simulink model "EMT_load"  (R2024a)
settings: Solver=ode1  StartTime=0.0  StopTime=simtime  FixedStep=Ts  RelTol=1e-3
values from neighbouring files (symbols this model uses):
  c0 = c0_hawk    (= 6.37282e-09)    [EMT_Phasor_parameters.m]
  c1 = c1_hawk    (= 8.76156e-09)    [EMT_Phasor_parameters.m]
  fg = 50    [EMT_Phasor_parameters.m]
  G1gen = 0.1245    [EMT_Phasor_parameters.m]
  G2gen = 0.30    (= 0.3)    [EMT_Phasor_parameters.m]
  G3gen = 0.20    (= 0.2)    [EMT_Phasor_parameters.m]
  G4sgen = 0.2078    [EMT_Phasor_parameters.m]
  G5gen = 0.20    (= 0.2)    [EMT_Phasor_parameters.m]
  G6gen = 0.2078    [EMT_Phasor_parameters.m]
  G6sgen = 0.20    (= 0.2)    [EMT_Phasor_parameters.m]
  G7gen = 0.518    [EMT_Phasor_parameters.m]
  Ihvpk = Ihv*sqrt(2)    [EMT_Phasor_parameters.m]
  l0 = l0_hawk    (= 0.00373)    [EMT_Phasor_parameters.m]
  l1 = l1_hawk    (= 0.00133)    [EMT_Phasor_parameters.m]
  L3dem = 0.10    (= 0.1)    [EMT_Phasor_parameters.m]
  L4dem = 0.30    (= 0.3)    [EMT_Phasor_parameters.m]
  L5dem = 0.35    [EMT_Phasor_parameters.m]
  L6dem = 0.15    [EMT_Phasor_parameters.m]
  L7dem = 0.10    (= 0.1)    [EMT_Phasor_parameters.m]
  Pr = Sr*PF    (= 550050000)    [EMT_Phasor_parameters.m]
  Qr = sqrt(Sr^2 - Pr^2)    [EMT_Phasor_parameters.m]
  r0 = r0_hawk    (= 0.44587)    [EMT_Phasor_parameters.m]
  r1 = r1_hawk    (= 0.12087)    [EMT_Phasor_parameters.m]
  Rtpu = Xtpu/40    (= 0.00375)    [EMT_Phasor_parameters.m]
  S1non = 400e6    (= 400000000)    [EMT_Phasor_parameters.m]
  S2non = 300e6    (= 300000000)    [EMT_Phasor_parameters.m]
  S3non = 200e6    (= 200000000)    [EMT_Phasor_parameters.m]
  S4snon = 200e6    (= 200000000)    [EMT_Phasor_parameters.m]
  S5non = 500e6    (= 500000000)    [EMT_Phasor_parameters.m]
  S6non = 400e6    (= 400000000)    [EMT_Phasor_parameters.m]
  S6snon = 200e6    (= 200000000)    [EMT_Phasor_parameters.m]
  S7non = 200e6    (= 200000000)    [EMT_Phasor_parameters.m]
  simtime = 5    [EMT_Phasor_parameters.m]
  tonvsc = 0.01    [EMT_Phasor_parameters.m]
  Ts = 150e-6    (= 0.00015)    [EMT_Phasor_parameters.m]
  Vhv = 220e3    (= 220000)    [EMT_Phasor_parameters.m]
  Vmv = 22e3    (= 22000)    [EMT_Phasor_parameters.m]
  wc1 = wsw1/10    (= 848.230016469)    [EMT_Phasor_parameters.m]
  wdc1 = wc1/10    (= 84.8230016469)    [EMT_Phasor_parameters.m]
  wpq1 = wc1/10    (= 84.8230016469)    [EMT_Phasor_parameters.m]
  wsw1 = ksw1*2*pi*fg    (= 8482.30016469)    [EMT_Phasor_parameters.m]
  Xtpu = 0.15    [EMT_Phasor_parameters.m]
undefined symbols (not defined in the file or in its folder): D11, Delta, Kf, r, theta0
libraries: simulink_extras x152, spsGroundLib x49, spsCurrentMeasurementLib x39, spsVoltageMeasurementLib x33, simulink x32, eeGeneralControl x32, slpidlib x32, powerlib x30, powerlib_meascontrol x28, spsFirstOrderFilterLib x24, eeTransforms x24, pid_lib x16
(part 6 of 16)

== system EMT_load/G2/VSC/VSC Control/Control loops/SW, EMT AVG, Phasor Quasi-EMT ==
  Pset : Inport
  Qset : Inport  Port=2
  vqd+- : Inport  Port=3
  iqd+- : Inport  Port=4
  freq : Inport  Port=5
  Block : Inport  Port=6
  Inner-loop : Subsystem
      settings: PortSchema="{\"entries\":[{\"content\":{\"sides\":[{\"content\":{\"connectorIds\":[\"In1\",\"In2\",\"In3\",\"In4\"]},\"type\":\"ConnectorPlacement.EquallySpacedRectSide\",\"uuid\":\"8a2e5096-891c-4956-8b6b-4b283c05b7bc\"},{\"content\":{\"connectorIds\":[\"Out1\",\"Out2\",\"Out3\",\"Out4\"],\"side\":\"RIGHT\"},\"type\":\"ConnectorPlacement.EquallySpacedRectSide\",\"uuid\":\"b7af4d2f-ce3f-4dc6-8323-535c80ee1784\"},{\"content\":{\"connectorIds\":[\"In5\",\"In6\",\"In7\"],\"side\":\"TOP\"},\"type\":\"ConnectorPlacement.EquallySpacedRectSide\",\"uuid\":\"1131cb27-465f-45b8-a6a1-03893285239a\"},{\"content\":{\"connectorIds\":[],\"side\":\"BOTTOM\"},\"type\":\"ConnectorPlacement.EquallySpacedRectSide\",\"uuid\":\"c84e74f4-9dae-42a7-97b7-61f404019883\"}]},\"type\":\"ConnectorPlacement.EquallySpacedConnector\",\"uuid\":\"8a900364-1293-46a0-8824-7b0f85f5a81c\"}],\"packageUris\":[\"http://schema.mathworks.com/mf0/Connector/19700101\"],\"version\":\"1.0\"}"
  Mux : Mux
  Outer-loop : Subsystem
      settings: PortSchema="{\"entries\":[{\"content\":{\"sides\":[{\"content\":{\"connectorIds\":[\"In1\",\"In2\",\"In3\",\"In4\",\"In5\"]},\"type\":\"ConnectorPlacement.EquallySpacedRectSide\",\"uuid\":\"9a334ab0-c6a2-41fb-a6ec-750715335523\"},{\"content\":{\"connectorIds\":[\"Out1\",\"Out2\",\"Out3\",\"Out4\",\"Out5\"],\"side\":\"RIGHT\"},\"type\":\"ConnectorPlacement.EquallySpacedRectSide\",\"uuid\":\"d3309230-0110-441f-b944-3d5d4312a42e\"},{\"content\":{\"connectorIds\":[\"In6\"],\"side\":\"TOP\"},\"type\":\"ConnectorPlacement.EquallySpacedRectSide\",\"uuid\":\"012603a1-4678-4ae1-91f6-3e17a1c8130b\"}]},\"type\":\"ConnectorPlacement.EquallySpacedConnector\",\"uuid\":\"299866d5-057c-44fe-b725-733ff7b8fc12\"}],\"packageUris\":[\"http://schema.mathworks.com/mf0/Connector/19700101\"],\"version\":\"1.0\"}"
  vqd+-ref : Outport
  m : Outport  Port=2
  wires:
  Mux/1 -> vqd+-ref/1
  Inner-loop/4(vd-*) -> Mux/4
  Inner-loop/3(vq-*) -> Mux/3
  Inner-loop/2(vd+*) -> Mux/2
  Inner-loop/1(vq+*) -> Mux/1
  Outer-loop/4(id-*) -> Inner-loop/4(id-*)
  Pset/1 -> Outer-loop/1(Pset)
  Qset/1 -> Outer-loop/2(Qset)
  Outer-loop/5(m) -> m/1
  Outer-loop/3(iq-*) -> Inner-loop/3(iq-*)
  freq/1 -> Outer-loop/5(freq)
  iqd+-/1 -> Inner-loop/7(iqd+-), Outer-loop/4(iqd+-)
  Block/1 -> Inner-loop/5(Blk), Outer-loop/6(Blk)
  vqd+-/1 -> Inner-loop/6(vqd+-), Outer-loop/3(vqd+-)
  Outer-loop/2(id+*) -> Inner-loop/2(id+*)
  Outer-loop/1(iq+*) -> Inner-loop/1(iq+*)

== system EMT_load/G2/VSC/VSC Control/Measurements/EMT ==
  note: abc to dq transformation
  Vabc : Inport
  Iabc : Inport  Port=2
  Gain2 : Gain  Gain=Vmv/Vhv
  Gain3 : Gain  Gain=Vhv/Vmv
  Iabc filter : spsFirstOrderFilterLib/First-Order Filter  Commented=through  FilterType=Lowpass  Tc=tfilt  Ts=0  Initialize=off  Vac_Init=[0, 0, 60]  Vdc_Init=0  PlotResponse=off  FreqRange="[0,  200,  1]"
  Mux : Mux
  Mux2 : Mux
  Mux3 : Mux  Inputs=2
  PLL aligned with positive-sequence : Subsystem
  Phase-sequence separation2 : Subsystem
  Phase-sequence separation3 : Subsystem
  "Power (3ph, Instantaneous)" : spsPower3phInstantaneousLib/Power (3ph, Instantaneous)
  Vabc filter : spsFirstOrderFilterLib/First-Order Filter  Commented=through  FilterType=Lowpass  Tc=tfilt  Ts=0  Initialize=off  Vac_Init=[0, 0, 60]  Vdc_Init=0  PlotResponse=off  FreqRange="[0,  200,  1]"
  freq : Outport
  theta : Outport  Port=2
  vqd+- : Outport  Port=3
  iqd+- : Outport  Port=4
  PQabc : Outport  Port=5
  wires:
  Phase-sequence separation2/2(d+) -> Mux/2
  Phase-sequence separation2/1(q+) -> Mux/1
  Iabc filter/1 -> Gain3/1
  Gain2/1 -> PLL aligned with positive-sequence/1(Vabc), Phase-sequence separation2/1(abc)
  Gain3/1 -> Phase-sequence separation3/1(abc)
  PLL aligned with positive-sequence/1(theta) -> Phase-sequence separation3/2(Theta), theta/1, Phase-sequence separation2/2(Theta)  "theta"
  PLL aligned with positive-sequence/2(f) -> freq/1
  Iabc/1 -> Iabc filter/1, [Iabc]
  Vabc filter/1 -> Gain2/1
  Vabc/1 -> Vabc filter/1, [Vabc]
  Mux/1 -> vqd+-/1  "vqd+-"
  Mux2/1 -> iqd+-/1  "iqd+-"
  Phase-sequence separation2/3(q-) -> Mux/3
  Phase-sequence separation2/4(d-) -> Mux/4
  Phase-sequence separation3/1(q+) -> Mux2/1
  Phase-sequence separation3/2(d+) -> Mux2/2
  Phase-sequence separation3/3(q-) -> Mux2/3
  Phase-sequence separation3/4(d-) -> Mux2/4
  "Power (3ph, Instantaneous)"/2 -> Mux3/2
  "Power (3ph, Instantaneous)"/1 -> Mux3/1
  Mux3/1 -> PQabc/1  "PQ1"
  [Iabc] -> "Power (3ph, Instantaneous)"/2
  [Vabc] -> "Power (3ph, Instantaneous)"/1

== system EMT_load/G2/VSC/VSC Control/Measurements/Phasor ==
  note: abc to dq transformation
      | (Phasor)
  Vabc : Inport
  Iabc : Inport  Port=2
  Complex to Magnitude-Angle : ComplexToMagnitudeAngle  Output=Angle
  Complex to Real-Imag{,1..3} (4 alike) : ComplexToRealImag
  Demux1 : Demux  Outputs=3
  Demux2 : Demux  Outputs=3
  Exp : Math  OutputSignalType=complex
  Frequency (Phasor)1 : Subsystem  mask{f0=fg, Ts=5e-3}
      mask prompts: f0 "Fundamental frequency (Hz)"; Ts "Derivative filter time constant (s)"
  Gain{,3..4,6..7} (5 alike) : Gain  Gain=-1
  Gain1 : Gain  Gain=Vhv/Vmv
  Gain2 : Gain  Gain=Vmv/Vhv
  Gain5 : Gain  Gain=-1i
  Instantaneous power (Phasor) : Subsystem
  Mux1 : Mux
  Mux2 : Mux
  Mux3 : Mux  Inputs=2
  Product{1..4} (4 alike) : Product
  Subsystem : Subsystem
      mask init:
      | a = exp(1i*2*pi/3);
      | a2 = exp(1i*4*pi/3);
  Subsystem1 : Subsystem
      mask init:
      | a = exp(1i*2*pi/3);
      | a2 = exp(1i*4*pi/3);
  Subsystem3 : Subsystem
      mask init:
      | a = exp(1i*2*pi/3);
      | a2 = exp(1i*4*pi/3);
  Terminator2 : Terminator
  Terminator4 : Terminator
  vqd+- : Outport
  iqd+- : Outport  Port=2
  freq : Outport  Port=3
  theta : Outport  Port=4
  PQabc : Outport  Port=5
  wires:
  Gain7/1 -> Mux2/4
  Gain6/1 -> Mux2/3
  Exp/1 -> Product1/1, Product4/1, Product2/2, Product3/2
  Product3/1 -> Complex to Real-Imag/1
  Demux2/2 -> Product3/1
  Demux2/3 -> Product2/1
  Gain5/1 -> Exp/1
  Complex to Magnitude-Angle/1 -> Frequency (Phasor)1/1(Phase), Gain5/1, theta/1  "theta"
  Product4/1 -> Complex to Real-Imag1/1
  Complex to Real-Imag/2 -> Mux1/2  "vd+"
  Demux1/3 -> Product1/2
  Demux1/2 -> Product4/2
  Subsystem/1(012) -> Demux2/1
  Demux2/1 -> Terminator2/1
  Demux1/1 -> Terminator4/1
  Subsystem1/1(012) -> Demux1/1
  Subsystem3/1(seq+) -> Complex to Magnitude-Angle/1
  Frequency (Phasor)1/1(Freq) -> freq/1
  Vabc/1 -> [Vabc], Gain2/1
  Gain2/1 -> Subsystem3/1(abc), Subsystem/1(abc)
  Product2/1 -> Complex to Real-Imag2/1
  Product1/1 -> Complex to Real-Imag3/1
  Mux1/1 -> vqd+-/1
  Complex to Real-Imag/1 -> Mux1/1  "vq+"
  Complex to Real-Imag2/1 -> Gain/1  "vq-"
  Complex to Real-Imag2/2 -> Gain3/1  "vd-"
  Complex to Real-Imag1/1 -> Mux2/1  "iq+"
  Complex to Real-Imag1/2 -> Gain4/1  "id+"
  Complex to Real-Imag3/1 -> Gain6/1  "iq-"
  Complex to Real-Imag3/2 -> Gain7/1  "id-"
  Mux2/1 -> iqd+-/1
  Iabc/1 -> [Iabc], Gain1/1
  Gain1/1 -> Subsystem1/1(abc)
  Gain/1 -> Mux1/3
  Gain3/1 -> Mux1/4
  Gain4/1 -> Mux2/2
  [Iabc] -> Instantaneous power (Phasor)/2(Iabc)
  Instantaneous power (Phasor)/2(Q) -> Mux3/2
  Instantaneous power (Phasor)/1(P) -> Mux3/1
  [Vabc] -> Instantaneous power (Phasor)/1(Vabc)
  Mux3/1 -> PQabc/1

== system EMT_load/G2/VSC/VSC Control/Modulation/EMT AVG ==
  note: Positive-sequence dq to abc
  note: Vref
  note: dq to abc
      | (AVG Model)
  note: negative-sequence dq to abc
  vqd+-* : Inport
  theta : Inport  Port=2
  Cartesian to Polar : simulink_extras/Transformations/Cartesian to Polar
  Cartesian to Polar1 : simulink_extras/Transformations/Cartesian to Polar
  Constant1 : Constant  Value=0
  Constant2 : Constant  Value=0
  Corrects delay : Subsystem
  Corrects delay1 : Subsystem
  Demux : Demux
  Gain : Gain  Gain=-1
  Gain2 : Gain  Gain=negseq_en
  Inverse Park Transform : eeTransforms/Inverse Park Transform  AxisAlignment=D-axis  PowerInvariant=off
  Inverse Park Transform1 : eeTransforms/Inverse Park Transform  AxisAlignment=D-axis  PowerInvariant=off
  Mux1 : Mux  Inputs=3
  Mux2 : Mux  Inputs=3
  Polar to Cartesian : simulink_extras/Transformations/Polar to Cartesian
  Polar to Cartesian1 : simulink_extras/Transformations/Polar to Cartesian
  Sum : Sum
  Sum1 : Sum  Inputs=|++
  Sum4 : Sum  Inputs=|++
  Unit Delay : UnitDelay  SampleTime=-1  HasFrameUpgradeWarning=on
  Ref : Outport
  wires:
  Demux/3 -> [vqnref]
  Demux/1 -> [vqpref]
  Demux/4 -> [vdnref]
  Demux/2 -> [vdpref]
  vqd+-*/1 -> Demux/1
  Gain2/1 -> Sum/2
  Polar to Cartesian/2 -> Mux1/2
  Sum4/1 -> Polar to Cartesian/2
  Mux1/1 -> Inverse Park Transform/1
  Cartesian to Polar/1 -> Polar to Cartesian/1
  [vdpref] -> Cartesian to Polar/1
  Cartesian to Polar/2 -> Sum4/1
  Constant1/1 -> Mux1/3
  [vqpref] -> Cartesian to Polar/2
  Corrects delay/1(dphi) -> Sum4/2
  Polar to Cartesian/1 -> Mux1/1
  Unit Delay/1 -> Ref/1
  [vdnref] -> Cartesian to Polar1/1
  Mux2/1 -> Inverse Park Transform1/1
  Cartesian to Polar1/1 -> Polar to Cartesian1/1
  Constant2/1 -> Mux2/3
  Polar to Cartesian1/2 -> Mux2/2
  Sum1/1 -> Polar to Cartesian1/2
  [vqnref] -> Cartesian to Polar1/2
  Corrects delay1/1(dphi) -> Sum1/2
  Gain/1 -> Inverse Park Transform1/2
  Polar to Cartesian1/1 -> Mux2/1
  Cartesian to Polar1/2 -> Sum1/1
  theta/1 -> Gain/1, Inverse Park Transform/2
  Sum/1 -> Unit Delay/1
  Inverse Park Transform/1 -> Sum/1
  Inverse Park Transform1/1 -> Gain2/1

== system EMT_load/G2/VSC/VSC Control/Modulation/EMT Switching ==
  note: Interpolate pulses
  note: Pulses
  note: Modulation
  note: negative-sequence dq to abc
  note: Positive-sequence dq to abc
  vqd+-* : Inport
  theta : Inport  Port=2
  Cartesian to Polar : simulink_extras/Transformations/Cartesian to Polar
  Cartesian to Polar1 : simulink_extras/Transformations/Cartesian to Polar
  Constant : Constant  Value=0
  Constant1 : Constant  Commented=on  Value=Vdc
  Constant2 : Constant  Value=0
  Corrects delay : Subsystem
  Corrects delay1 : Subsystem
  Demux : Demux
  Gain : Gain  Gain=1/(Vdc/2)
  Gain1 : Gain  Gain=-1
  Gain2 : Gain  Gain=negseq_en
  Inverse Park Transform1 : eeTransforms/Inverse Park Transform  AxisAlignment=D-axis  PowerInvariant=off
  Inverse Park Transform2 : eeTransforms/Inverse Park Transform  AxisAlignment=D-axis  PowerInvariant=off
  Mux : Mux  Inputs=3
  Mux1 : Mux  Inputs=3
  Mux2 : Mux  Inputs=3
  PWM Generator (Interpolation)1 : powerlib_meascontrol/Pulse & Signal Generators/PWM Generator (Interpolation)  GeneratorType=Two-level, three-phase  Fc=ksw*fg  InitialPhase=0  Ts=Ts
  "PWM Generator (Three-phase, Two-level)" : eePwmGeneratorTwoLevel/PWM Generator (Three-phase, Two-level)  Commented=on  PWMMode=Continuous PWM (CPWM)  CPWMMode=SPWM: sinusoidal PWM  DPWMMode=60 DPWM: 60 degree discontinuous PWM  fsw=ksw*fg  Ts=Ts
  Polar to Cartesian : simulink_extras/Transformations/Polar to Cartesian
  Polar to Cartesian1 : simulink_extras/Transformations/Polar to Cartesian
  Sum : Sum
  Sum1 : Sum  Inputs=|++
  Sum4 : Sum  Inputs=|++
  Unit Delay : UnitDelay  SampleTime=-1  HasFrameUpgradeWarning=on
  Ref : Outport
  wires:
  [vqpref] -> Cartesian to Polar/2
  Demux/4 -> [vdnref]
  Demux/3 -> [vqnref]
  Demux/2 -> [vdpref]
  Demux/1 -> [vqpref]
  vqd+-*/1 -> Demux/1
  Mux1/1 -> Unit Delay/1
  Sum/1 -> Gain/1
  Unit Delay/1 -> Ref/1
  PWM Generator (Interpolation)1/2 -> Mux1/2
  PWM Generator (Interpolation)1/1 -> Mux1/1
  PWM Generator (Interpolation)1/3 -> Mux1/3
  Gain/1 -> PWM Generator (Interpolation)1/1
  Constant1/1 -> "PWM Generator (Three-phase, Two-level)"/2
  theta/1 -> Inverse Park Transform2/2, Gain1/1
  Gain2/1 -> Sum/2
  Constant/1 -> Mux/3
  Cartesian to Polar/2 -> Sum4/1
  Sum4/1 -> Polar to Cartesian/2
  Corrects delay/1(dphi) -> Sum4/2
  Cartesian to Polar/1 -> Polar to Cartesian/1
  Mux/1 -> Inverse Park Transform2/1
  Polar to Cartesian/1 -> Mux/1
  Polar to Cartesian/2 -> Mux/2
  [vdpref] -> Cartesian to Polar/1
  Mux2/1 -> Inverse Park Transform1/1
  Sum1/1 -> Polar to Cartesian1/2
  Inverse Park Transform2/1 -> Sum/1
  Corrects delay1/1(dphi) -> Sum1/2
  Polar to Cartesian1/2 -> Mux2/2
  Cartesian to Polar1/1 -> Polar to Cartesian1/1
  Cartesian to Polar1/2 -> Sum1/1
  Polar to Cartesian1/1 -> Mux2/1
  [vdnref] -> Cartesian to Polar1/1
  [vqnref] -> Cartesian to Polar1/2
  Inverse Park Transform1/1 -> Gain2/1
  Constant2/1 -> Mux2/3
  Gain1/1 -> Inverse Park Transform1/2

== system EMT_load/G2/VSC/VSC Control/Modulation/Phasor I and Phasor PQ ==
  note: Negative-sequence dq to abc
  note: Positive-sequence dq to abc
  note: dq to abc
      | (Phasor I and Phasor PQ)
  iqd+-* : Inport
  theta : Inport  Port=2
  Constant : Constant  Commented=on  Value=negseq_en
  Constant1 : Constant  Value=complex(0,0)
  Delay : Delay  DelayLength=1
  Demux3 : Demux
  Display : Display  Commented=on
  Exp : Math  OutputSignalType=complex
  Exp1 : Math  OutputSignalType=complex
  Gain : Gain  Gain=-1
  Gain1 : Gain  Gain=1i
  Gain2 : Gain  Gain=exp(1i*pi/6)
  Gain3 : Gain  Gain=exp(-1i*pi/6)
  Gain5 : Gain  Gain=1i
  Gain7 : Gain  Gain=negseq_en
  Gain8 : Gain  Gain=-1
  Gain9 : Gain  Gain=-1
  Inverse Park Transform (Phasor) : Subsystem  Commented=on
  Mux3 : Mux  Inputs=3
  Product : Product
  Product1 : Product
  RL time constant : Subsystem  Commented=through  mask{R=Rt, L=Lt, f=fg}
      mask prompts: R "Series resistance (R)"; L "Series inductance (L)"; f "Power frequency (Hz)"
      mask init:
      | w = 2*pi*f;
  Real-Imag to Complex : RealImagToComplex
  Real-Imag to Complex1 : RealImagToComplex
  Subsystem : Subsystem
      mask init:
      | a = exp(1i*2*pi/3);
      | a2 = exp(1i*4*pi/3);
  Ref : Outport
  wires:
  Demux3/4 -> [idnref]
  iqd+-*/1 -> Demux3/1
  Demux3/1 -> [iqpref]
  Demux3/2 -> [idpref]
  Demux3/3 -> [iqnref]
  Constant/1 -> Display/1
  Gain/1 -> Real-Imag to Complex/2
  [idpref] -> Gain/1
  Exp1/1 -> Product1/1
  Real-Imag to Complex1/1 -> Product1/2
  Gain1/1 -> Exp1/1
  Constant1/1 -> Mux3/1
  Mux3/1 -> Subsystem/1(012)
  Product/1 -> Gain2/1
  Real-Imag to Complex/1 -> Product/1
  [iqpref] -> Real-Imag to Complex/1
  Exp/1 -> Product/2
  Gain5/1 -> Exp/1
  theta/1 -> Gain1/1, Gain5/1
  Delay/1 -> Ref/1
  Subsystem/1(abc) -> Delay/1
  Gain3/1 -> Mux3/3
  Product1/1 -> Gain7/1
  Gain7/1 -> Gain3/1
  [idnref] -> Gain8/1
  [iqnref] -> Gain9/1
  Gain9/1 -> Real-Imag to Complex1/1
  Gain8/1 -> Real-Imag to Complex1/2
  Gain2/1 -> Mux3/2

== system EMT_load/G2/VSC/VSC Control/Modulation/Phasor Quasi-EMT ==
  note: dq to abc
      | (Phasor)
  note: Positive-sequence dq to abc
  note: Negative-sequence dq to abc
  vqd+-* : Inport
  theta : Inport  Port=2
  vqd+- : Inport  Port=3
  Cartesian to Polar : simulink_extras/Transformations/Cartesian to Polar
  Cartesian to Polar1 : simulink_extras/Transformations/Cartesian to Polar
  Constant : Constant  Commented=on  Value=negseq_en
  Constant1 : Constant  Value=complex(0,0)
  Corrects delay : Subsystem  Commented=on
  Corrects delay2 : Subsystem  Commented=on
  Delay : Delay  DelayLength=1
  Demux : Demux  Outputs=2
  Demux1 : Demux  Outputs=2
  Demux2 : Demux
  Demux3 : Demux
  Display : Display  Commented=on
  Exp : Math  OutputSignalType=complex
  Exp1 : Math  OutputSignalType=complex
  Gain : Gain  Gain=-1
  Gain1 : Gain  Gain=1i
  Gain2 : Gain  Gain=exp(1i*pi/6)
  Gain3 : Gain  Gain=exp(-1i*pi/6)
  Gain5 : Gain  Gain=1i
  Gain7 : Gain  Gain=negseq_en
  Gain8 : Gain  Gain=-1
  Gain9 : Gain  Gain=-1
  Inverse Park Transform (Phasor) : Subsystem  Commented=on
  Mux{,1..2,4} (4 alike) : Mux  Inputs=2
  Mux3 : Mux  Inputs=3
  Polar to Cartesian : simulink_extras/Transformations/Polar to Cartesian
  Polar to Cartesian1 : simulink_extras/Transformations/Polar to Cartesian
  Product : Product
  Product1 : Product
  Real-Imag to Complex : RealImagToComplex
  Real-Imag to Complex1 : RealImagToComplex
  Subsystem : Subsystem
      mask init:
      | a = exp(1i*2*pi/3);
      | a2 = exp(1i*4*pi/3);
  Sum1 : Sum  Inputs=|++
  Sum4 : Sum  Inputs=|++
  V to I RL (+seq) : Subsystem  mask{R=Rt, L=Lt, f=fg}
      mask prompts: R "Series resistance (R)"; L "Series inductance (L)"; f "Power frequency (Hz)"
      mask init:
      | w = 2*pi*f;
  V to I RL (- seq) : Subsystem  mask{R=Rt, L=Lt, f=fg}
      mask prompts: R "Series resistance (R)"; L "Series inductance (L)"; f "Power frequency (Hz)"
      mask init:
      | w = 2*pi*f;
  Ref : Outport
  wires:
  Demux3/3 -> [vqnref]
  Demux3/4 -> [vdnref]
  Demux3/1 -> [vqpref]
  vqd+-*/1 -> Demux3/1
  Demux3/2 -> [vdpref]
  Gain2/1 -> Mux3/2
  Gain8/1 -> Real-Imag to Complex1/2
  Gain9/1 -> Real-Imag to Complex1/1
  Demux1/2 -> Gain9/1
  Demux1/1 -> Gain8/1
  Gain7/1 -> Gain3/1
  Product1/1 -> Gain7/1
  Gain3/1 -> Mux3/3
  Subsystem/1(abc) -> Delay/1
  Delay/1 -> Ref/1
  Cartesian to Polar1/1 -> Polar to Cartesian1/1
  theta/1 -> Gain5/1, Gain1/1
  [vqp] -> Mux1/2
  V to I RL (+seq)/1(idIq) -> Demux/1
  Gain5/1 -> Exp/1
  Exp/1 -> Product/2
  Demux/2 -> Real-Imag to Complex/1
  Real-Imag to Complex/1 -> Product/1
  Product/1 -> Gain2/1
  Mux3/1 -> Subsystem/1(012)
  Constant1/1 -> Mux3/1
  Sum4/1 -> Polar to Cartesian/2
  Cartesian to Polar/1 -> Polar to Cartesian/1
  Cartesian to Polar/2 -> Sum4/1
  Corrects delay/1(dphi) -> Sum4/2
  Polar to Cartesian/1 -> Mux/1
  Polar to Cartesian/2 -> Mux/2
  [vdpref] -> Cartesian to Polar/1
  [vqpref] -> Cartesian to Polar/2
  Mux/1 -> V to I RL (+seq)/2(Vdq2)
  Mux1/1 -> V to I RL (+seq)/1(Vdq1)
  [vdnref] -> Cartesian to Polar1/1
  Sum1/1 -> Polar to Cartesian1/2
  [vqnref] -> Cartesian to Polar1/2
  Polar to Cartesian1/2 -> Mux2/2
  Polar to Cartesian1/1 -> Mux2/1
  Cartesian to Polar1/2 -> Sum1/1
  Corrects delay2/1(dphi) -> Sum1/2
  Mux2/1 -> V to I RL (- seq)/2(Vdq2)
  Mux4/1 -> V to I RL (- seq)/1(Vdq1)
  [vqn] -> Mux4/2
  [vdn] -> Mux4/1
  V to I RL (- seq)/1(idIq) -> Demux1/1
  Gain1/1 -> Exp1/1
  Real-Imag to Complex1/1 -> Product1/2
  Exp1/1 -> Product1/1
  vqd+-/1 -> Demux2/1
  Demux2/2 -> [vdp]
  Demux2/3 -> [vqn]
  Demux2/4 -> [vdn]
  Demux2/1 -> [vqp]
  [vdp] -> Mux1/1
  Demux/1 -> Gain/1
  Gain/1 -> Real-Imag to Complex/2
  Constant/1 -> Display/1

== system EMT_load/G3/VSC/VSC Control/Control loops/Phasor I 1st ==
  Pset : Inport
  Qset : Inport  Port=2
  vqd+- : Inport  Port=3
  iqd+- : Inport  Port=4
  freq : Inport  Port=5
  Block : Inport  Port=6
  Inner-loop : Subsystem
  Mux : Mux
  Outer-loop : Subsystem
      settings: PortSchema="{\"entries\":[{\"content\":{\"sides\":[{\"content\":{\"connectorIds\":[\"In1\",\"In2\",\"In3\",\"In4\",\"In5\"]},\"type\":\"ConnectorPlacement.EquallySpacedRectSide\",\"uuid\":\"9a334ab0-c6a2-41fb-a6ec-750715335523\"},{\"content\":{\"connectorIds\":[\"Out1\",\"Out2\",\"Out3\",\"Out4\",\"Out5\"],\"side\":\"RIGHT\"},\"type\":\"ConnectorPlacement.EquallySpacedRectSide\",\"uuid\":\"d3309230-0110-441f-b944-3d5d4312a42e\"},{\"content\":{\"connectorIds\":[\"In6\"],\"side\":\"TOP\"},\"type\":\"ConnectorPlacement.EquallySpacedRectSide\",\"uuid\":\"012603a1-4678-4ae1-91f6-3e17a1c8130b\"}]},\"type\":\"ConnectorPlacement.EquallySpacedConnector\",\"uuid\":\"299866d5-057c-44fe-b725-733ff7b8fc12\"}],\"packageUris\":[\"http://schema.mathworks.com/mf0/Connector/19700101\"],\"version\":\"1.0\"}"
  iqd+-ref : Outport
  m : Outport  Port=2
  wires:
  Outer-loop/4(id-*) -> Inner-loop/4(id-*)
  Outer-loop/3(iq-*) -> Inner-loop/3(iq-*)
  Outer-loop/2(id+*) -> Inner-loop/2(id+*)
  Outer-loop/1(iq+*) -> Inner-loop/1(iq+*)
  Block/1 -> Outer-loop/6(Blk)
  vqd+-/1 -> Outer-loop/3(vqd+-)
  freq/1 -> Outer-loop/5(freq)
  iqd+-/1 -> Outer-loop/4(iqd+-)
  Inner-loop/2(id+ref) -> Mux/2
  Pset/1 -> Outer-loop/1(Pset)
  Outer-loop/5(m) -> m/1
  Qset/1 -> Outer-loop/2(Qset)
  Mux/1 -> iqd+-ref/1
  Inner-loop/3(iq-ref) -> Mux/3
  Inner-loop/1(iq+ref) -> Mux/1
  Inner-loop/4(id-ref) -> Mux/4

== system EMT_load/G3/VSC/VSC Control/Control loops/Phasor I ref ==
  Pset : Inport
  Qset : Inport  Port=2
  vqd+- : Inport  Port=3
  iqd+- : Inport  Port=4
  freq : Inport  Port=5
  Block : Inport  Port=6
  Mux : Mux
  Outer-loop : Subsystem
      settings: PortSchema="{\"entries\":[{\"content\":{\"sides\":[{\"content\":{\"connectorIds\":[\"In1\",\"In2\",\"In3\",\"In4\",\"In5\"]},\"type\":\"ConnectorPlacement.EquallySpacedRectSide\",\"uuid\":\"9a334ab0-c6a2-41fb-a6ec-750715335523\"},{\"content\":{\"connectorIds\":[\"Out1\",\"Out2\",\"Out3\",\"Out4\",\"Out5\"],\"side\":\"RIGHT\"},\"type\":\"ConnectorPlacement.EquallySpacedRectSide\",\"uuid\":\"d3309230-0110-441f-b944-3d5d4312a42e\"},{\"content\":{\"connectorIds\":[\"In6\"],\"side\":\"TOP\"},\"type\":\"ConnectorPlacement.EquallySpacedRectSide\",\"uuid\":\"012603a1-4678-4ae1-91f6-3e17a1c8130b\"}]},\"type\":\"ConnectorPlacement.EquallySpacedConnector\",\"uuid\":\"299866d5-057c-44fe-b725-733ff7b8fc12\"}],\"packageUris\":[\"http://schema.mathworks.com/mf0/Connector/19700101\"],\"version\":\"1.0\"}"
  iqd+-ref : Outport
  m : Outport  Port=2
  wires:
  Outer-loop/4(id-*) -> Mux/4
  Outer-loop/1(iq+*) -> Mux/1
  Outer-loop/3(iq-*) -> Mux/3
  Mux/1 -> iqd+-ref/1
  Qset/1 -> Outer-loop/2(Qset)
  Outer-loop/5(m) -> m/1
  Pset/1 -> Outer-loop/1(Pset)
  Outer-loop/2(id+*) -> Mux/2
  iqd+-/1 -> Outer-loop/4(iqd+-)
  freq/1 -> Outer-loop/5(freq)
  vqd+-/1 -> Outer-loop/3(vqd+-)
  Block/1 -> Outer-loop/6(Blk)

== system EMT_load/G3/VSC/VSC Control/Control loops/Phasor PQ 1st ==
  Pset : Inport
  Qset : Inport  Port=2
  vqd+- : Inport  Port=3
  iqd+- : Inport  Port=4
  freq : Inport  Port=5
  Block : Inport  Port=6
  Mux : Mux
  Outer-loop : Subsystem
      settings: PortSchema="{\"entries\":[{\"content\":{\"sides\":[{\"content\":{\"connectorIds\":[\"In1\",\"In2\",\"In3\",\"In4\",\"In5\"]},\"type\":\"ConnectorPlacement.EquallySpacedRectSide\",\"uuid\":\"9a334ab0-c6a2-41fb-a6ec-750715335523\"},{\"content\":{\"connectorIds\":[\"Out1\",\"Out2\",\"Out3\",\"Out4\",\"Out5\"],\"side\":\"RIGHT\"},\"type\":\"ConnectorPlacement.EquallySpacedRectSide\",\"uuid\":\"d3309230-0110-441f-b944-3d5d4312a42e\"},{\"content\":{\"connectorIds\":[\"In6\"],\"side\":\"TOP\"},\"type\":\"ConnectorPlacement.EquallySpacedRectSide\",\"uuid\":\"012603a1-4678-4ae1-91f6-3e17a1c8130b\"}]},\"type\":\"ConnectorPlacement.EquallySpacedConnector\",\"uuid\":\"299866d5-057c-44fe-b725-733ff7b8fc12\"}],\"packageUris\":[\"http://schema.mathworks.com/mf0/Connector/19700101\"],\"version\":\"1.0\"}"
  iqd+-ref : Outport
  m : Outport  Port=2
  wires:
  Block/1 -> Outer-loop/6(Blk)
  vqd+-/1 -> Outer-loop/3(vqd+-)
  freq/1 -> Outer-loop/5(freq)
  iqd+-/1 -> Outer-loop/4(iqd+-)
  Outer-loop/2(id+*) -> Mux/2
  Pset/1 -> Outer-loop/1(Pset)
  Outer-loop/5(m) -> m/1
  Qset/1 -> Outer-loop/2(Qset)
  Mux/1 -> iqd+-ref/1
  Outer-loop/3(iq-*) -> Mux/3
  Outer-loop/1(iq+*) -> Mux/1
  Outer-loop/4(id-*) -> Mux/4

== system EMT_load/G3/VSC/VSC Control/Control loops/SW, EMT AVG, Phasor Quasi-EMT ==
  Pset : Inport
  Qset : Inport  Port=2
  vqd+- : Inport  Port=3
  iqd+- : Inport  Port=4
  freq : Inport  Port=5
  Block : Inport  Port=6
  Inner-loop : Subsystem
      settings: PortSchema="{\"entries\":[{\"content\":{\"sides\":[{\"content\":{\"connectorIds\":[\"In1\",\"In2\",\"In3\",\"In4\"]},\"type\":\"ConnectorPlacement.EquallySpacedRectSide\",\"uuid\":\"8a2e5096-891c-4956-8b6b-4b283c05b7bc\"},{\"content\":{\"connectorIds\":[\"Out1\",\"Out2\",\"Out3\",\"Out4\"],\"side\":\"RIGHT\"},\"type\":\"ConnectorPlacement.EquallySpacedRectSide\",\"uuid\":\"b7af4d2f-ce3f-4dc6-8323-535c80ee1784\"},{\"content\":{\"connectorIds\":[\"In5\",\"In6\",\"In7\"],\"side\":\"TOP\"},\"type\":\"ConnectorPlacement.EquallySpacedRectSide\",\"uuid\":\"1131cb27-465f-45b8-a6a1-03893285239a\"},{\"content\":{\"connectorIds\":[],\"side\":\"BOTTOM\"},\"type\":\"ConnectorPlacement.EquallySpacedRectSide\",\"uuid\":\"c84e74f4-9dae-42a7-97b7-61f404019883\"}]},\"type\":\"ConnectorPlacement.EquallySpacedConnector\",\"uuid\":\"8a900364-1293-46a0-8824-7b0f85f5a81c\"}],\"packageUris\":[\"http://schema.mathworks.com/mf0/Connector/19700101\"],\"version\":\"1.0\"}"
  Mux : Mux
  Outer-loop : Subsystem
      settings: PortSchema="{\"entries\":[{\"content\":{\"sides\":[{\"content\":{\"connectorIds\":[\"In1\",\"In2\",\"In3\",\"In4\",\"In5\"]},\"type\":\"ConnectorPlacement.EquallySpacedRectSide\",\"uuid\":\"9a334ab0-c6a2-41fb-a6ec-750715335523\"},{\"content\":{\"connectorIds\":[\"Out1\",\"Out2\",\"Out3\",\"Out4\",\"Out5\"],\"side\":\"RIGHT\"},\"type\":\"ConnectorPlacement.EquallySpacedRectSide\",\"uuid\":\"d3309230-0110-441f-b944-3d5d4312a42e\"},{\"content\":{\"connectorIds\":[\"In6\"],\"side\":\"TOP\"},\"type\":\"ConnectorPlacement.EquallySpacedRectSide\",\"uuid\":\"012603a1-4678-4ae1-91f6-3e17a1c8130b\"}]},\"type\":\"ConnectorPlacement.EquallySpacedConnector\",\"uuid\":\"299866d5-057c-44fe-b725-733ff7b8fc12\"}],\"packageUris\":[\"http://schema.mathworks.com/mf0/Connector/19700101\"],\"version\":\"1.0\"}"
  vqd+-ref : Outport
  m : Outport  Port=2
  wires:
  Mux/1 -> vqd+-ref/1
  Inner-loop/4(vd-*) -> Mux/4
  Inner-loop/3(vq-*) -> Mux/3
  Inner-loop/2(vd+*) -> Mux/2
  Inner-loop/1(vq+*) -> Mux/1
  Outer-loop/4(id-*) -> Inner-loop/4(id-*)
  Pset/1 -> Outer-loop/1(Pset)
  Qset/1 -> Outer-loop/2(Qset)
  Outer-loop/5(m) -> m/1
  Outer-loop/3(iq-*) -> Inner-loop/3(iq-*)
  freq/1 -> Outer-loop/5(freq)
  iqd+-/1 -> Inner-loop/7(iqd+-), Outer-loop/4(iqd+-)
  Block/1 -> Inner-loop/5(Blk), Outer-loop/6(Blk)
  vqd+-/1 -> Inner-loop/6(vqd+-), Outer-loop/3(vqd+-)
  Outer-loop/2(id+*) -> Inner-loop/2(id+*)
  Outer-loop/1(iq+*) -> Inner-loop/1(iq+*)

== system EMT_load/G3/VSC/VSC Control/Measurements/EMT ==
  note: abc to dq transformation
  Vabc : Inport
  Iabc : Inport  Port=2
  Gain2 : Gain  Gain=Vmv/Vhv
  Gain3 : Gain  Gain=Vhv/Vmv
  Iabc filter : spsFirstOrderFilterLib/First-Order Filter  Commented=through  FilterType=Lowpass  Tc=tfilt  Ts=0  Initialize=off  Vac_Init=[0, 0, 60]  Vdc_Init=0  PlotResponse=off  FreqRange="[0,  200,  1]"
  Mux : Mux
  Mux2 : Mux
  Mux3 : Mux  Inputs=2
  PLL aligned with positive-sequence : Subsystem
  Phase-sequence separation2 : Subsystem
  Phase-sequence separation3 : Subsystem
  "Power (3ph, Instantaneous)" : spsPower3phInstantaneousLib/Power (3ph, Instantaneous)
  Vabc filter : spsFirstOrderFilterLib/First-Order Filter  Commented=through  FilterType=Lowpass  Tc=tfilt  Ts=0  Initialize=off  Vac_Init=[0, 0, 60]  Vdc_Init=0  PlotResponse=off  FreqRange="[0,  200,  1]"
  freq : Outport
  theta : Outport  Port=2
  vqd+- : Outport  Port=3
  iqd+- : Outport  Port=4
  PQabc : Outport  Port=5
  wires:
  Phase-sequence separation2/2(d+) -> Mux/2
  Phase-sequence separation2/1(q+) -> Mux/1
  Iabc filter/1 -> Gain3/1
  Gain2/1 -> PLL aligned with positive-sequence/1(Vabc), Phase-sequence separation2/1(abc)
  Gain3/1 -> Phase-sequence separation3/1(abc)
  PLL aligned with positive-sequence/1(theta) -> Phase-sequence separation3/2(Theta), theta/1, Phase-sequence separation2/2(Theta)  "theta"
  PLL aligned with positive-sequence/2(f) -> freq/1
  Iabc/1 -> Iabc filter/1, [Iabc]
  Vabc filter/1 -> Gain2/1
  Vabc/1 -> Vabc filter/1, [Vabc]
  Mux/1 -> vqd+-/1  "vqd+-"
  Mux2/1 -> iqd+-/1  "iqd+-"
  Phase-sequence separation2/3(q-) -> Mux/3
  Phase-sequence separation2/4(d-) -> Mux/4
  Phase-sequence separation3/1(q+) -> Mux2/1
  Phase-sequence separation3/2(d+) -> Mux2/2
  Phase-sequence separation3/3(q-) -> Mux2/3
  Phase-sequence separation3/4(d-) -> Mux2/4
  "Power (3ph, Instantaneous)"/2 -> Mux3/2
  "Power (3ph, Instantaneous)"/1 -> Mux3/1
  Mux3/1 -> PQabc/1  "PQ1"
  [Iabc] -> "Power (3ph, Instantaneous)"/2
  [Vabc] -> "Power (3ph, Instantaneous)"/1

== system EMT_load/G3/VSC/VSC Control/Measurements/Phasor ==
  note: abc to dq transformation
      | (Phasor)
  Vabc : Inport
  Iabc : Inport  Port=2
  Complex to Magnitude-Angle : ComplexToMagnitudeAngle  Output=Angle
  Complex to Real-Imag{,1..3} (4 alike) : ComplexToRealImag
  Demux1 : Demux  Outputs=3
  Demux2 : Demux  Outputs=3
  Exp : Math  OutputSignalType=complex
  Frequency (Phasor)1 : Subsystem  mask{f0=fg, Ts=5e-3}
      mask prompts: f0 "Fundamental frequency (Hz)"; Ts "Derivative filter time constant (s)"
  Gain{,3..4,6..7} (5 alike) : Gain  Gain=-1
  Gain1 : Gain  Gain=Vhv/Vmv
  Gain2 : Gain  Gain=Vmv/Vhv
  Gain5 : Gain  Gain=-1i
  Instantaneous power (Phasor) : Subsystem
  Mux1 : Mux
  Mux2 : Mux
  Mux3 : Mux  Inputs=2
  Product{1..4} (4 alike) : Product
  Subsystem : Subsystem
      mask init:
      | a = exp(1i*2*pi/3);
      | a2 = exp(1i*4*pi/3);
  Subsystem1 : Subsystem
      mask init:
      | a = exp(1i*2*pi/3);
      | a2 = exp(1i*4*pi/3);
  Subsystem3 : Subsystem
      mask init:
      | a = exp(1i*2*pi/3);
      | a2 = exp(1i*4*pi/3);
  Terminator2 : Terminator
  Terminator4 : Terminator
  vqd+- : Outport
  iqd+- : Outport  Port=2
  freq : Outport  Port=3
  theta : Outport  Port=4
  PQabc : Outport  Port=5
  wires:
  Gain7/1 -> Mux2/4
  Gain6/1 -> Mux2/3
  Exp/1 -> Product1/1, Product4/1, Product2/2, Product3/2
  Product3/1 -> Complex to Real-Imag/1
  Demux2/2 -> Product3/1
  Demux2/3 -> Product2/1
  Gain5/1 -> Exp/1
  Complex to Magnitude-Angle/1 -> Frequency (Phasor)1/1(Phase), Gain5/1, theta/1  "theta"
  Product4/1 -> Complex to Real-Imag1/1
  Complex to Real-Imag/2 -> Mux1/2  "vd+"
  Demux1/3 -> Product1/2
  Demux1/2 -> Product4/2
  Subsystem/1(012) -> Demux2/1
  Demux2/1 -> Terminator2/1
  Demux1/1 -> Terminator4/1
  Subsystem1/1(012) -> Demux1/1
  Subsystem3/1(seq+) -> Complex to Magnitude-Angle/1
  Frequency (Phasor)1/1(Freq) -> freq/1
  Vabc/1 -> [Vabc], Gain2/1
  Gain2/1 -> Subsystem3/1(abc), Subsystem/1(abc)
  Product2/1 -> Complex to Real-Imag2/1
  Product1/1 -> Complex to Real-Imag3/1
  Mux1/1 -> vqd+-/1
  Complex to Real-Imag/1 -> Mux1/1  "vq+"
  Complex to Real-Imag2/1 -> Gain/1  "vq-"
  Complex to Real-Imag2/2 -> Gain3/1  "vd-"
  Complex to Real-Imag1/1 -> Mux2/1  "iq+"
  Complex to Real-Imag1/2 -> Gain4/1  "id+"
  Complex to Real-Imag3/1 -> Gain6/1  "iq-"
  Complex to Real-Imag3/2 -> Gain7/1  "id-"
  Mux2/1 -> iqd+-/1
  Iabc/1 -> [Iabc], Gain1/1
  Gain1/1 -> Subsystem1/1(abc)
  Gain/1 -> Mux1/3
  Gain3/1 -> Mux1/4
  Gain4/1 -> Mux2/2
  [Iabc] -> Instantaneous power (Phasor)/2(Iabc)
  Instantaneous power (Phasor)/2(Q) -> Mux3/2
  Instantaneous power (Phasor)/1(P) -> Mux3/1
  [Vabc] -> Instantaneous power (Phasor)/1(Vabc)
  Mux3/1 -> PQabc/1

== system EMT_load/G3/VSC/VSC Control/Modulation/EMT AVG ==
  note: Positive-sequence dq to abc
  note: Vref
  note: dq to abc
      | (AVG Model)
  note: negative-sequence dq to abc
  vqd+-* : Inport
  theta : Inport  Port=2
  Cartesian to Polar : simulink_extras/Transformations/Cartesian to Polar
  Cartesian to Polar1 : simulink_extras/Transformations/Cartesian to Polar
  Constant1 : Constant  Value=0
  Constant2 : Constant  Value=0
  Corrects delay : Subsystem
  Corrects delay1 : Subsystem
  Demux : Demux
  Gain : Gain  Gain=-1
  Gain2 : Gain  Gain=negseq_en
  Inverse Park Transform : eeTransforms/Inverse Park Transform  AxisAlignment=D-axis  PowerInvariant=off
  Inverse Park Transform1 : eeTransforms/Inverse Park Transform  AxisAlignment=D-axis  PowerInvariant=off
  Mux1 : Mux  Inputs=3
  Mux2 : Mux  Inputs=3
  Polar to Cartesian : simulink_extras/Transformations/Polar to Cartesian
  Polar to Cartesian1 : simulink_extras/Transformations/Polar to Cartesian
  Sum : Sum
  Sum1 : Sum  Inputs=|++
  Sum4 : Sum  Inputs=|++
  Unit Delay : UnitDelay  SampleTime=-1  HasFrameUpgradeWarning=on
  Ref : Outport
  wires:
  Demux/3 -> [vqnref]
  Demux/1 -> [vqpref]
  Demux/4 -> [vdnref]
  Demux/2 -> [vdpref]
  vqd+-*/1 -> Demux/1
  Gain2/1 -> Sum/2
  Polar to Cartesian/2 -> Mux1/2
  Sum4/1 -> Polar to Cartesian/2
  Mux1/1 -> Inverse Park Transform/1
  Cartesian to Polar/1 -> Polar to Cartesian/1
  [vdpref] -> Cartesian to Polar/1
  Cartesian to Polar/2 -> Sum4/1
  Constant1/1 -> Mux1/3
  [vqpref] -> Cartesian to Polar/2
  Corrects delay/1(dphi) -> Sum4/2
  Polar to Cartesian/1 -> Mux1/1
  Unit Delay/1 -> Ref/1
  [vdnref] -> Cartesian to Polar1/1
  Mux2/1 -> Inverse Park Transform1/1
  Cartesian to Polar1/1 -> Polar to Cartesian1/1
  Constant2/1 -> Mux2/3
  Polar to Cartesian1/2 -> Mux2/2
  Sum1/1 -> Polar to Cartesian1/2
  [vqnref] -> Cartesian to Polar1/2
  Corrects delay1/1(dphi) -> Sum1/2
  Gain/1 -> Inverse Park Transform1/2
  Polar to Cartesian1/1 -> Mux2/1
  Cartesian to Polar1/2 -> Sum1/1
  theta/1 -> Gain/1, Inverse Park Transform/2
  Sum/1 -> Unit Delay/1
  Inverse Park Transform/1 -> Sum/1
  Inverse Park Transform1/1 -> Gain2/1

== system EMT_load/G3/VSC/VSC Control/Modulation/EMT Switching ==
  note: Interpolate pulses
  note: Pulses
  note: Modulation
  note: negative-sequence dq to abc
  note: Positive-sequence dq to abc
  vqd+-* : Inport
  theta : Inport  Port=2
  Cartesian to Polar : simulink_extras/Transformations/Cartesian to Polar
  Cartesian to Polar1 : simulink_extras/Transformations/Cartesian to Polar
  Constant : Constant  Value=0
  Constant1 : Constant  Commented=on  Value=Vdc
  Constant2 : Constant  Value=0
  Corrects delay : Subsystem
  Corrects delay1 : Subsystem
  Demux : Demux
  Gain : Gain  Gain=1/(Vdc/2)
  Gain1 : Gain  Gain=-1
  Gain2 : Gain  Gain=negseq_en
  Inverse Park Transform1 : eeTransforms/Inverse Park Transform  AxisAlignment=D-axis  PowerInvariant=off
  Inverse Park Transform2 : eeTransforms/Inverse Park Transform  AxisAlignment=D-axis  PowerInvariant=off
  Mux : Mux  Inputs=3
  Mux1 : Mux  Inputs=3
  Mux2 : Mux  Inputs=3
  PWM Generator (Interpolation)1 : powerlib_meascontrol/Pulse & Signal Generators/PWM Generator (Interpolation)  GeneratorType=Two-level, three-phase  Fc=ksw*fg  InitialPhase=0  Ts=Ts
  "PWM Generator (Three-phase, Two-level)" : eePwmGeneratorTwoLevel/PWM Generator (Three-phase, Two-level)  Commented=on  PWMMode=Continuous PWM (CPWM)  CPWMMode=SPWM: sinusoidal PWM  DPWMMode=60 DPWM: 60 degree discontinuous PWM  fsw=ksw*fg  Ts=Ts
  Polar to Cartesian : simulink_extras/Transformations/Polar to Cartesian
  Polar to Cartesian1 : simulink_extras/Transformations/Polar to Cartesian
  Sum : Sum
  Sum1 : Sum  Inputs=|++
  Sum4 : Sum  Inputs=|++
  Unit Delay : UnitDelay  SampleTime=-1  HasFrameUpgradeWarning=on
  Ref : Outport
  wires:
  [vqpref] -> Cartesian to Polar/2
  Demux/4 -> [vdnref]
  Demux/3 -> [vqnref]
  Demux/2 -> [vdpref]
  Demux/1 -> [vqpref]
  vqd+-*/1 -> Demux/1
  Mux1/1 -> Unit Delay/1
  Sum/1 -> Gain/1
  Unit Delay/1 -> Ref/1
  PWM Generator (Interpolation)1/2 -> Mux1/2
  PWM Generator (Interpolation)1/1 -> Mux1/1
  PWM Generator (Interpolation)1/3 -> Mux1/3
  Gain/1 -> PWM Generator (Interpolation)1/1
  Constant1/1 -> "PWM Generator (Three-phase, Two-level)"/2
  theta/1 -> Inverse Park Transform2/2, Gain1/1
  Gain2/1 -> Sum/2
  Constant/1 -> Mux/3
  Cartesian to Polar/2 -> Sum4/1
  Sum4/1 -> Polar to Cartesian/2
  Corrects delay/1(dphi) -> Sum4/2
  Cartesian to Polar/1 -> Polar to Cartesian/1
  Mux/1 -> Inverse Park Transform2/1
  Polar to Cartesian/1 -> Mux/1
  Polar to Cartesian/2 -> Mux/2
  [vdpref] -> Cartesian to Polar/1
  Mux2/1 -> Inverse Park Transform1/1
  Sum1/1 -> Polar to Cartesian1/2
  Inverse Park Transform2/1 -> Sum/1
  Corrects delay1/1(dphi) -> Sum1/2
  Polar to Cartesian1/2 -> Mux2/2
  Cartesian to Polar1/1 -> Polar to Cartesian1/1
  Cartesian to Polar1/2 -> Sum1/1
  Polar to Cartesian1/1 -> Mux2/1
  [vdnref] -> Cartesian to Polar1/1
  [vqnref] -> Cartesian to Polar1/2
  Inverse Park Transform1/1 -> Gain2/1
  Constant2/1 -> Mux2/3
  Gain1/1 -> Inverse Park Transform1/2

== system EMT_load/G3/VSC/VSC Control/Modulation/Phasor I and Phasor PQ ==
  note: Negative-sequence dq to abc
  note: Positive-sequence dq to abc
  note: dq to abc
      | (Phasor I and Phasor PQ)
  iqd+-* : Inport
  theta : Inport  Port=2
  Constant : Constant  Commented=on  Value=negseq_en
  Constant1 : Constant  Value=complex(0,0)
  Delay : Delay  DelayLength=1
  Demux3 : Demux
  Display : Display  Commented=on
  Exp : Math  OutputSignalType=complex
  Exp1 : Math  OutputSignalType=complex
  Gain : Gain  Gain=-1
  Gain1 : Gain  Gain=1i
  Gain2 : Gain  Gain=exp(1i*pi/6)
  Gain3 : Gain  Gain=exp(-1i*pi/6)
  Gain5 : Gain  Gain=1i
  Gain7 : Gain  Gain=negseq_en
  Gain8 : Gain  Gain=-1
  Gain9 : Gain  Gain=-1
  Inverse Park Transform (Phasor) : Subsystem  Commented=on
  Mux3 : Mux  Inputs=3
  Product : Product
  Product1 : Product
  RL time constant : Subsystem  Commented=through  mask{R=Rt, L=Lt, f=fg}
      mask prompts: R "Series resistance (R)"; L "Series inductance (L)"; f "Power frequency (Hz)"
      mask init:
      | w = 2*pi*f;
  Real-Imag to Complex : RealImagToComplex
  Real-Imag to Complex1 : RealImagToComplex
  Subsystem : Subsystem
      mask init:
      | a = exp(1i*2*pi/3);
      | a2 = exp(1i*4*pi/3);
  Ref : Outport
  wires:
  Demux3/4 -> [idnref]
  iqd+-*/1 -> Demux3/1
  Demux3/1 -> [iqpref]
  Demux3/2 -> [idpref]
  Demux3/3 -> [iqnref]
  Constant/1 -> Display/1
  Gain/1 -> Real-Imag to Complex/2
  [idpref] -> Gain/1
  Exp1/1 -> Product1/1
  Real-Imag to Complex1/1 -> Product1/2
  Gain1/1 -> Exp1/1
  Constant1/1 -> Mux3/1
  Mux3/1 -> Subsystem/1(012)
  Product/1 -> Gain2/1
  Real-Imag to Complex/1 -> Product/1
  [iqpref] -> Real-Imag to Complex/1
  Exp/1 -> Product/2
  Gain5/1 -> Exp/1
  theta/1 -> Gain1/1, Gain5/1
  Delay/1 -> Ref/1
  Subsystem/1(abc) -> Delay/1
  Gain3/1 -> Mux3/3
  Product1/1 -> Gain7/1
  Gain7/1 -> Gain3/1
  [idnref] -> Gain8/1
  [iqnref] -> Gain9/1
  Gain9/1 -> Real-Imag to Complex1/1
  Gain8/1 -> Real-Imag to Complex1/2
  Gain2/1 -> Mux3/2

== system EMT_load/G3/VSC/VSC Control/Modulation/Phasor Quasi-EMT ==
  note: dq to abc
      | (Phasor)
  note: Positive-sequence dq to abc
  note: Negative-sequence dq to abc
  vqd+-* : Inport
  theta : Inport  Port=2
  vqd+- : Inport  Port=3
  Cartesian to Polar : simulink_extras/Transformations/Cartesian to Polar
  Cartesian to Polar1 : simulink_extras/Transformations/Cartesian to Polar
  Constant : Constant  Commented=on  Value=negseq_en
  Constant1 : Constant  Value=complex(0,0)
  Corrects delay : Subsystem  Commented=on
  Corrects delay2 : Subsystem  Commented=on
  Delay : Delay  DelayLength=1
  Demux : Demux  Outputs=2
  Demux1 : Demux  Outputs=2
  Demux2 : Demux
  Demux3 : Demux
  Display : Display  Commented=on
  Exp : Math  OutputSignalType=complex
  Exp1 : Math  OutputSignalType=complex
  Gain : Gain  Gain=-1
  Gain1 : Gain  Gain=1i
  Gain2 : Gain  Gain=exp(1i*pi/6)
  Gain3 : Gain  Gain=exp(-1i*pi/6)
  Gain5 : Gain  Gain=1i
  Gain7 : Gain  Gain=negseq_en
  Gain8 : Gain  Gain=-1
  Gain9 : Gain  Gain=-1
  Inverse Park Transform (Phasor) : Subsystem  Commented=on
  Mux{,1..2,4} (4 alike) : Mux  Inputs=2
  Mux3 : Mux  Inputs=3
  Polar to Cartesian : simulink_extras/Transformations/Polar to Cartesian
  Polar to Cartesian1 : simulink_extras/Transformations/Polar to Cartesian
  Product : Product
  Product1 : Product
  Real-Imag to Complex : RealImagToComplex
  Real-Imag to Complex1 : RealImagToComplex
  Subsystem : Subsystem
      mask init:
      | a = exp(1i*2*pi/3);
      | a2 = exp(1i*4*pi/3);
  Sum1 : Sum  Inputs=|++
  Sum4 : Sum  Inputs=|++
  V to I RL (+seq) : Subsystem  mask{R=Rt, L=Lt, f=fg}
      mask prompts: R "Series resistance (R)"; L "Series inductance (L)"; f "Power frequency (Hz)"
      mask init:
      | w = 2*pi*f;
  V to I RL (- seq) : Subsystem  mask{R=Rt, L=Lt, f=fg}
      mask prompts: R "Series resistance (R)"; L "Series inductance (L)"; f "Power frequency (Hz)"
      mask init:
      | w = 2*pi*f;
  Ref : Outport
  wires:
  Demux3/3 -> [vqnref]
  Demux3/4 -> [vdnref]
  Demux3/1 -> [vqpref]
  vqd+-*/1 -> Demux3/1
  Demux3/2 -> [vdpref]
  Gain2/1 -> Mux3/2
  Gain8/1 -> Real-Imag to Complex1/2
  Gain9/1 -> Real-Imag to Complex1/1
  Demux1/2 -> Gain9/1
  Demux1/1 -> Gain8/1
  Gain7/1 -> Gain3/1
  Product1/1 -> Gain7/1
  Gain3/1 -> Mux3/3
  Subsystem/1(abc) -> Delay/1
  Delay/1 -> Ref/1
  Cartesian to Polar1/1 -> Polar to Cartesian1/1
  theta/1 -> Gain5/1, Gain1/1
  [vqp] -> Mux1/2
  V to I RL (+seq)/1(idIq) -> Demux/1
  Gain5/1 -> Exp/1
  Exp/1 -> Product/2
  Demux/2 -> Real-Imag to Complex/1
  Real-Imag to Complex/1 -> Product/1
  Product/1 -> Gain2/1
  Mux3/1 -> Subsystem/1(012)
  Constant1/1 -> Mux3/1
  Sum4/1 -> Polar to Cartesian/2
  Cartesian to Polar/1 -> Polar to Cartesian/1
  Cartesian to Polar/2 -> Sum4/1
  Corrects delay/1(dphi) -> Sum4/2
  Polar to Cartesian/1 -> Mux/1
  Polar to Cartesian/2 -> Mux/2
  [vdpref] -> Cartesian to Polar/1
  [vqpref] -> Cartesian to Polar/2
  Mux/1 -> V to I RL (+seq)/2(Vdq2)
  Mux1/1 -> V to I RL (+seq)/1(Vdq1)
  [vdnref] -> Cartesian to Polar1/1
  Sum1/1 -> Polar to Cartesian1/2
  [vqnref] -> Cartesian to Polar1/2
  Polar to Cartesian1/2 -> Mux2/2
  Polar to Cartesian1/1 -> Mux2/1
  Cartesian to Polar1/2 -> Sum1/1
  Corrects delay2/1(dphi) -> Sum1/2
  Mux2/1 -> V to I RL (- seq)/2(Vdq2)
  Mux4/1 -> V to I RL (- seq)/1(Vdq1)
  [vqn] -> Mux4/2
  [vdn] -> Mux4/1
  V to I RL (- seq)/1(idIq) -> Demux1/1
  Gain1/1 -> Exp1/1
  Real-Imag to Complex1/1 -> Product1/2
  Exp1/1 -> Product1/1
  vqd+-/1 -> Demux2/1
  Demux2/2 -> [vdp]
  Demux2/3 -> [vqn]
  Demux2/4 -> [vdn]
  Demux2/1 -> [vqp]
  [vdp] -> Mux1/1
  Demux/1 -> Gain/1
  Gain/1 -> Real-Imag to Complex/2
  Constant/1 -> Display/1

== system EMT_load/G5/VSC/VSC Control/Control loops/Phasor I 1st ==
  Pset : Inport
  Qset : Inport  Port=2
  vqd+- : Inport  Port=3
  iqd+- : Inport  Port=4
  freq : Inport  Port=5
  Block : Inport  Port=6
  Inner-loop : Subsystem
  Mux : Mux
  Outer-loop : Subsystem
      settings: PortSchema="{\"entries\":[{\"content\":{\"sides\":[{\"content\":{\"connectorIds\":[\"In1\",\"In2\",\"In3\",\"In4\",\"In5\"]},\"type\":\"ConnectorPlacement.EquallySpacedRectSide\",\"uuid\":\"9a334ab0-c6a2-41fb-a6ec-750715335523\"},{\"content\":{\"connectorIds\":[\"Out1\",\"Out2\",\"Out3\",\"Out4\",\"Out5\"],\"side\":\"RIGHT\"},\"type\":\"ConnectorPlacement.EquallySpacedRectSide\",\"uuid\":\"d3309230-0110-441f-b944-3d5d4312a42e\"},{\"content\":{\"connectorIds\":[\"In6\"],\"side\":\"TOP\"},\"type\":\"ConnectorPlacement.EquallySpacedRectSide\",\"uuid\":\"012603a1-4678-4ae1-91f6-3e17a1c8130b\"}]},\"type\":\"ConnectorPlacement.EquallySpacedConnector\",\"uuid\":\"299866d5-057c-44fe-b725-733ff7b8fc12\"}],\"packageUris\":[\"http://schema.mathworks.com/mf0/Connector/19700101\"],\"version\":\"1.0\"}"
  iqd+-ref : Outport
  m : Outport  Port=2
  wires:
  Outer-loop/4(id-*) -> Inner-loop/4(id-*)
  Outer-loop/3(iq-*) -> Inner-loop/3(iq-*)
  Outer-loop/2(id+*) -> Inner-loop/2(id+*)
  Outer-loop/1(iq+*) -> Inner-loop/1(iq+*)
  Block/1 -> Outer-loop/6(Blk)
  vqd+-/1 -> Outer-loop/3(vqd+-)
  freq/1 -> Outer-loop/5(freq)
  iqd+-/1 -> Outer-loop/4(iqd+-)
  Inner-loop/2(id+ref) -> Mux/2
  Pset/1 -> Outer-loop/1(Pset)
  Outer-loop/5(m) -> m/1
  Qset/1 -> Outer-loop/2(Qset)
  Mux/1 -> iqd+-ref/1
  Inner-loop/3(iq-ref) -> Mux/3
  Inner-loop/1(iq+ref) -> Mux/1
  Inner-loop/4(id-ref) -> Mux/4

== system EMT_load/G5/VSC/VSC Control/Control loops/Phasor I ref ==
  Pset : Inport
  Qset : Inport  Port=2
  vqd+- : Inport  Port=3
  iqd+- : Inport  Port=4
  freq : Inport  Port=5
  Block : Inport  Port=6
  Mux : Mux
  Outer-loop : Subsystem
      settings: PortSchema="{\"entries\":[{\"content\":{\"sides\":[{\"content\":{\"connectorIds\":[\"In1\",\"In2\",\"In3\",\"In4\",\"In5\"]},\"type\":\"ConnectorPlacement.EquallySpacedRectSide\",\"uuid\":\"9a334ab0-c6a2-41fb-a6ec-750715335523\"},{\"content\":{\"connectorIds\":[\"Out1\",\"Out2\",\"Out3\",\"Out4\",\"Out5\"],\"side\":\"RIGHT\"},\"type\":\"ConnectorPlacement.EquallySpacedRectSide\",\"uuid\":\"d3309230-0110-441f-b944-3d5d4312a42e\"},{\"content\":{\"connectorIds\":[\"In6\"],\"side\":\"TOP\"},\"type\":\"ConnectorPlacement.EquallySpacedRectSide\",\"uuid\":\"012603a1-4678-4ae1-91f6-3e17a1c8130b\"}]},\"type\":\"ConnectorPlacement.EquallySpacedConnector\",\"uuid\":\"299866d5-057c-44fe-b725-733ff7b8fc12\"}],\"packageUris\":[\"http://schema.mathworks.com/mf0/Connector/19700101\"],\"version\":\"1.0\"}"
  iqd+-ref : Outport
  m : Outport  Port=2
  wires:
  Outer-loop/4(id-*) -> Mux/4
  Outer-loop/1(iq+*) -> Mux/1
  Outer-loop/3(iq-*) -> Mux/3
  Mux/1 -> iqd+-ref/1
  Qset/1 -> Outer-loop/2(Qset)
  Outer-loop/5(m) -> m/1
  Pset/1 -> Outer-loop/1(Pset)
  Outer-loop/2(id+*) -> Mux/2
  iqd+-/1 -> Outer-loop/4(iqd+-)
  freq/1 -> Outer-loop/5(freq)
  vqd+-/1 -> Outer-loop/3(vqd+-)
  Block/1 -> Outer-loop/6(Blk)

== system EMT_load/G5/VSC/VSC Control/Control loops/Phasor PQ 1st ==
  Pset : Inport
  Qset : Inport  Port=2
  vqd+- : Inport  Port=3
  iqd+- : Inport  Port=4
  freq : Inport  Port=5
  Block : Inport  Port=6
  Mux : Mux
  Outer-loop : Subsystem
      settings: PortSchema="{\"entries\":[{\"content\":{\"sides\":[{\"content\":{\"connectorIds\":[\"In1\",\"In2\",\"In3\",\"In4\",\"In5\"]},\"type\":\"ConnectorPlacement.EquallySpacedRectSide\",\"uuid\":\"9a334ab0-c6a2-41fb-a6ec-750715335523\"},{\"content\":{\"connectorIds\":[\"Out1\",\"Out2\",\"Out3\",\"Out4\",\"Out5\"],\"side\":\"RIGHT\"},\"type\":\"ConnectorPlacement.EquallySpacedRectSide\",\"uuid\":\"d3309230-0110-441f-b944-3d5d4312a42e\"},{\"content\":{\"connectorIds\":[\"In6\"],\"side\":\"TOP\"},\"type\":\"ConnectorPlacement.EquallySpacedRectSide\",\"uuid\":\"012603a1-4678-4ae1-91f6-3e17a1c8130b\"}]},\"type\":\"ConnectorPlacement.EquallySpacedConnector\",\"uuid\":\"299866d5-057c-44fe-b725-733ff7b8fc12\"}],\"packageUris\":[\"http://schema.mathworks.com/mf0/Connector/19700101\"],\"version\":\"1.0\"}"
  iqd+-ref : Outport
  m : Outport  Port=2
  wires:
  Block/1 -> Outer-loop/6(Blk)
  vqd+-/1 -> Outer-loop/3(vqd+-)
  freq/1 -> Outer-loop/5(freq)
  iqd+-/1 -> Outer-loop/4(iqd+-)
  Outer-loop/2(id+*) -> Mux/2
  Pset/1 -> Outer-loop/1(Pset)
  Outer-loop/5(m) -> m/1
  Qset/1 -> Outer-loop/2(Qset)
  Mux/1 -> iqd+-ref/1
  Outer-loop/3(iq-*) -> Mux/3
  Outer-loop/1(iq+*) -> Mux/1
  Outer-loop/4(id-*) -> Mux/4
